simulink model "AsyncBoost"  (R2021a)
settings: Solver=VariableStepAuto  StartTime=0.0  StopTime=10.0  RelTol=1e-3
undefined symbols (not defined in the file or in its folder): plecs
settings Model: Creator=dcostine  LastModifiedBy=dcostine

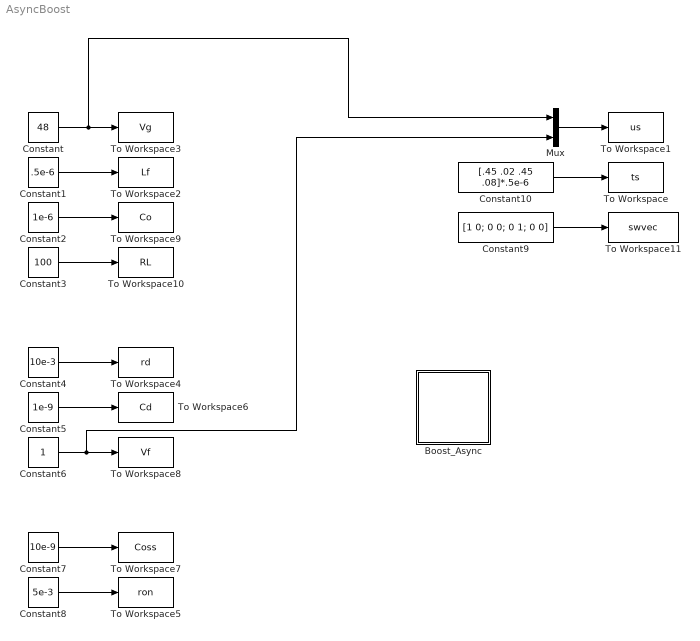
== system AsyncBoost ==
  Boost_Async : Subsystem  LoadFcn=plecs('sl', 200);  InitFcn=plecs('sl', 214);  StartFcn=plecs('sl', 208);  StopFcn=plecs('sl', 209);  mask(PlecsCircuit){PLECSData=<binary blob, 1804 chars, not shown>}
      mask prompts: PLECSData "PLECS Data (Do not delete or modify!)"
      mask init:
      | % PLACE CUSTOM INITIALIZATIONS ABOVE
      | % DO NOT REMOVE
      | plecs('sl', 215);
      | % DO NOT REMOVE
      settings: CopyFcn=plecs('sl', 203);  DeleteFcn=plecs('sl', 205);  UndoDeleteFcn=plecs('sl', 206);  PreSaveFcn=plecs('sl', 211);  PostSaveFcn=plecs('sl', 201);  NameChangeFcn=plecs('sl', 210);  DestroyFcn=plecs('sl', 207);  PreCopyFcn=plecs('sl', 216);  OpenFcn=plecs('sl', 202);  ErrorFcn=plerrorfcn
      mask Help: web(['file:///' fullfile(plecsdoc, 'creatingacircuit.html')])
      mask Display: disp('PLECS\nCircuit')
  Constant : Constant  Value=48
  Constant1 : Constant  Value=.5e-6
  Constant10 : Constant  Value=[.45 .02 .45 .08]*.5e-6
  Constant2 : Constant  Value=1e-6
  Constant3 : Constant  Value=100
  Constant4 : Constant  Value=10e-3
  Constant5 : Constant  Value=1e-9
  Constant6 : Constant
  Constant7 : Constant  Value=10e-9
  Constant8 : Constant  Value=5e-3
  Constant9 : Constant  Value=[1 0; 0 0; 0 1; 0 0]
  Mux : Mux  Inputs=2
  To Workspace : ToWorkspace  VariableName=ts  SampleTime=-1
  To Workspace1 : ToWorkspace  VariableName=us  SampleTime=-1
  To Workspace10 : ToWorkspace  VariableName=RL  SampleTime=-1
  To Workspace11 : ToWorkspace  VariableName=swvec  SampleTime=-1
  To Workspace2 : ToWorkspace  VariableName=Lf  SampleTime=-1
  To Workspace3 : ToWorkspace  VariableName=Vg  SampleTime=-1
  To Workspace4 : ToWorkspace  VariableName=rd  SampleTime=-1
  To Workspace5 : ToWorkspace  VariableName=ron  SampleTime=-1
  To Workspace6 : ToWorkspace  VariableName=Cd  SampleTime=-1
  To Workspace7 : ToWorkspace  VariableName=Coss  SampleTime=-1
  To Workspace8 : ToWorkspace  VariableName=Vf  SampleTime=-1
  To Workspace9 : ToWorkspace  VariableName=Co  SampleTime=-1
  wires:
  Constant1/1 -> To Workspace2/1
  Constant2/1 -> To Workspace9/1
  Constant3/1 -> To Workspace10/1
  Constant5/1 -> To Workspace6/1
  Constant4/1 -> To Workspace4/1
  Constant6/1 -> Mux/2, To Workspace8/1
  Constant7/1 -> To Workspace7/1
  Constant8/1 -> To Workspace5/1
  Constant/1 -> Mux/1, To Workspace3/1
  Constant10/1 -> To Workspace/1
  Constant9/1 -> To Workspace11/1
  Mux/1 -> To Workspace1/1

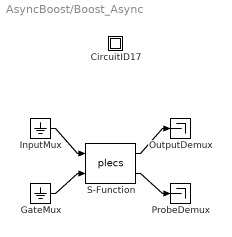
== system AsyncBoost/Boost_Async ==
  " CircuitID17 " : Subsystem
  " GateMux " : Ground
  " InputMux " : Ground
  " OutputDemux " : Terminator
  " ProbeDemux " : Terminator
  " S-Function " : S-Function  FunctionName=plecs  SFunctionDeploymentMode=off  EnableBusSupport=off
  wires:
  " InputMux "/1 -> " S-Function "/1
  " GateMux "/1 -> " S-Function "/2
  " S-Function "/1 -> " OutputDemux "/1
  " S-Function "/2 -> " ProbeDemux "/1

== system AsyncBoost/Boost_Async/ CircuitID17  ==
